simulink model "k_First_Order_Thermal_System"  (R2024b)
settings: Solver=VariableStepAuto  StartTime=0.0  StopTime=100  RelTol=1e-3
settings Model: Creator=Hp  LastModifiedBy=Hp

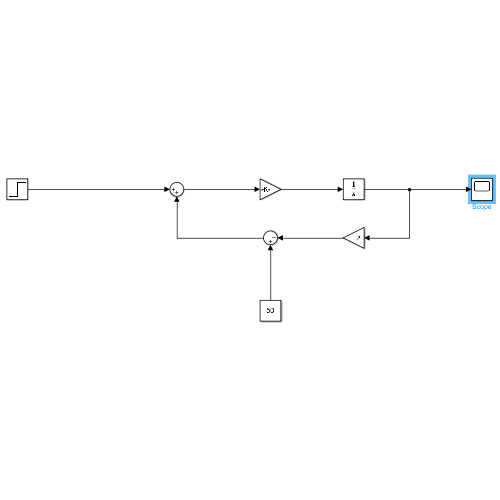
[thumbnail: Simulink's stored preview of the top-level diagram]
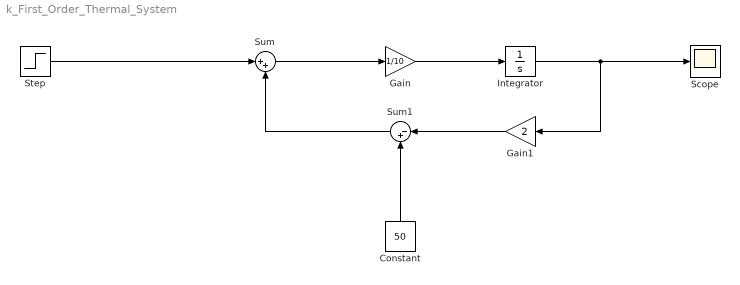
== system k_First_Order_Thermal_System ==
  Constant : Constant  Value=50
  Gain : Gain  Gain=1/10
  Gain1 : Gain  Gain=2
  Integrator : Integrator  InitialCondition=25
  Scope : Scope
  Step : Step  Time=0  After=100  SampleTime=0
  Sum : Sum  Inputs=|++
  Sum1 : Sum  Inputs=|-+
  wires:
  Integrator/1 -> Gain1/1, Scope/1
  Step/1 -> Sum/1
  Sum/1 -> Gain/1
  Gain/1 -> Integrator/1
  Gain1/1 -> Sum1/1
  Constant/1 -> Sum1/2
  Sum1/1 -> Sum/2
